simulink model "sampleModel313"  (R2021b)
settings: Solver=VariableStepAuto  StartTime=0.0  StopTime=10.0  RelTol=1e-3
undefined symbols (not defined in the file or in its folder): Newton, Raphson
libraries: simulink x5, slpidlib x1
settings Model: Creator=user  LastModifiedBy=user

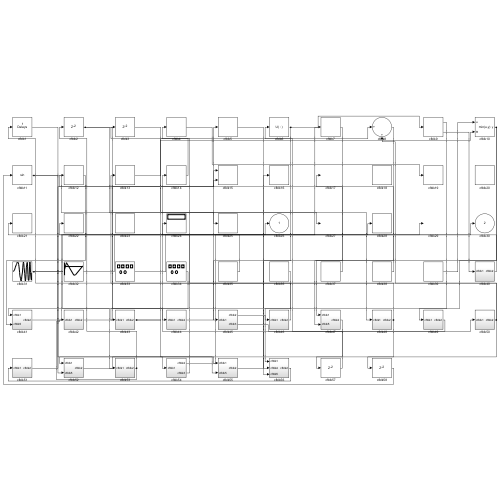
[thumbnail: Simulink's stored preview of the top-level diagram]
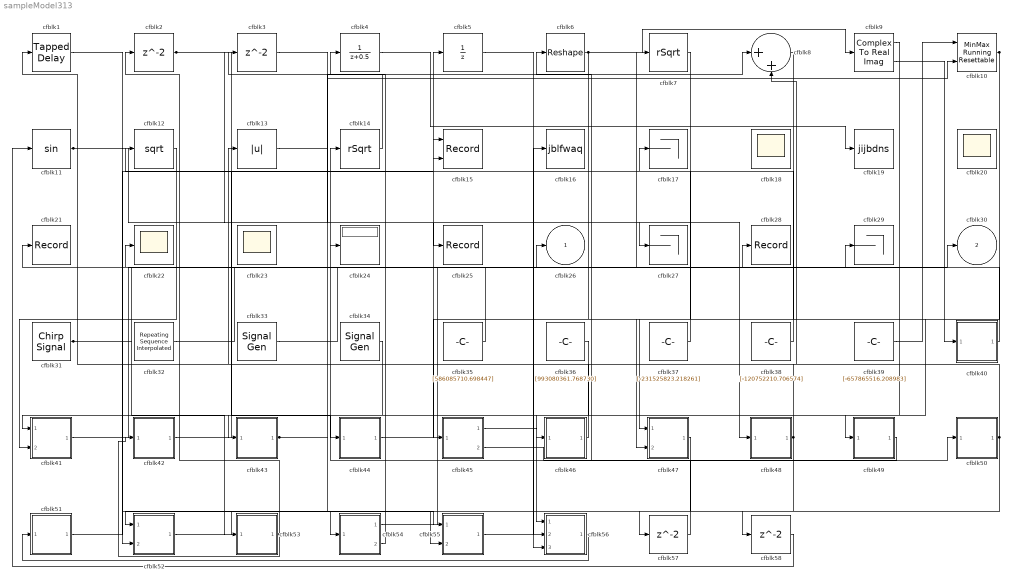
== system sampleModel313 ==
  cfblk1 : simulink/Discrete/Tapped Delay  vinit=0.0  samptime=-1  NumDelays=1  DelayOrder=Oldest  includeCurrent=off
  cfblk10 : simulink/Math Operations/MinMax Running Resettable  Function=min  vinit=0.0
  cfblk11 : Trigonometry
  cfblk12 : Sqrt  SaturateOnIntegerOverflow=on
  cfblk13 : Abs
  cfblk14 : Sqrt  Operator=rSqrt  AlgorithmType=Newton-Raphson  SaturateOnIntegerOverflow=on
  cfblk15 : Record  FileSettingsInternal="{\"entries\":[{\"content\":{\"excelSettings\":{\"content\":{},\"type\":\"Streamout.ExcelSettings\"}},\"type\":\"Streamout.FileSettingStorage\",\"uuid\":\"90899390-830c-4f20-99b3-b71a0b28f61d\"}],\"packageUris\":[\"http://schema.mathworks.com/mf0/streamout_blocks/R2020a\"],\"version\":\"1.0\"}"  Layout=[1 1]  SignalsInternal="{\"entries\":[{\"content\":{\"signals\":[{\"content\":{\"blockPath\":[\"sampleModel313/cfblk15\"],\"channel\":[],\"dimensions\":[1],\"domain\":\"sampleModel313/cfblk15\",\"lineColor\":\"#a2142f\",\"plots\":[1],\"port\":1,\"sid\":[\"\"],\"signalID\":13225,\"signalName\":\"cfblk42\"},\"type\":\"RecordBlkView.Signal\",\"uuid\":\"8692cdac-150e-44d6-933d-60e6954af18a\"},{\"content\":{\"blockPath\":[\"sampleModel313/cfblk15\"],\"channel\":[],\"dimensions\":[1],\"domain\":\"sampleModel313/cfblk15\",\"lineColor\":\"#139fff\",\"plots\":[1],\"port\":2,\"sid\":[\"\"],\"signalID\":13229,\"signalName\":\"cfblk51\"},\"type\":\"RecordBlkView.Signal\",\"uuid\":\"bc72ad84-1dd7-4dd2-a75b-1e74ba305bc3\"}]},\"type\":\"RecordBlkView.InputSignals\",\"uuid\":\"f9261edf-1019-4a70-a12e-24402ee5b183\"}],\"packageUris\":[\"http://schema.mathworks.com/mf0/streamout_blocks/R2020a\"],\"version\":\"1.0\"}"  VisualizationBindings="{\"xyplotplugin\":{\"info\":[{\"series\":[{\"bindingParametersList\":[{\"parameter\":\"X-Axis\",\"signalID\":13225,\"signalName\":\"cfblk42\"},{\"parameter\":\"Y-Axis\",\"signalID\":13229,\"signalName\":\"cfblk51\"}],\"seriesID\":56227}],\"subplotID\":1}]}}"  CompatibilityTag=XY
  cfblk16 : ToWorkspace  VariableName=jblfwaq  SaveFormat=Timeseries  SampleTime=-1
  cfblk17 : Terminator
  cfblk{18,20,22..23} (4 alike) : Scope
      cfblk18 settings: Floating=on
      cfblk20 settings: Floating=on
      cfblk23 settings: Floating=on
  cfblk19 : ToWorkspace  VariableName=jijbdns  SaveFormat=Timeseries  SampleTime=-1
  cfblk{2..3,57..58} (4 alike) : Delay  SampleTime=1
  cfblk21 : Record  FileSettingsInternal="{\"entries\":[{\"content\":{\"excelSettings\":{\"content\":{},\"type\":\"Streamout.ExcelSettings\"}},\"type\":\"Streamout.FileSettingStorage\",\"uuid\":\"64d57652-56fd-4ca2-b7c9-7809ea16690a\"}],\"packageUris\":[\"http://schema.mathworks.com/mf0/streamout_blocks/R2020a\"],\"version\":\"1.0\"}"  SignalsInternal="{\"entries\":[{\"content\":{\"signals\":[{\"content\":{\"blockPath\":[\"sampleModel313/cfblk21\"],\"channel\":[],\"dimensions\":[1],\"domain\":\"sampleModel313/cfblk21\",\"lineColor\":\"#d95319\",\"plots\":[1],\"port\":1,\"sid\":[\"\"],\"signalID\":13233,\"signalName\":\"cfblk54:2\"},\"type\":\"RecordBlkView.Signal\",\"uuid\":\"e54faf43-b919-4a37-b4a8-d819c38ad15e\"}]},\"type\":\"RecordBlkView.InputSignals\",\"uuid\":\"55d9d209-326f-41d9-bd73-887f268fbcdd\"}],\"packageUris\":[\"http://schema.mathworks.com/mf0/streamout_blocks/R2020a\"],\"version\":\"1.0\"}"  VisualizationBindings="{\"sparklinesplugin\":{\"info\":[{\"bindingParametersList\":[],\"subplotID\":1}]}}"
  cfblk24 : Display
  cfblk25 : Record  FileSettingsInternal="{\"entries\":[{\"content\":{\"excelSettings\":{\"content\":{},\"type\":\"Streamout.ExcelSettings\"}},\"type\":\"Streamout.FileSettingStorage\",\"uuid\":\"0e3c709e-7826-4611-a778-3b371a044123\"}],\"packageUris\":[\"http://schema.mathworks.com/mf0/streamout_blocks/R2020a\"],\"version\":\"1.0\"}"  SignalsInternal="{\"entries\":[{\"content\":{\"signals\":[{\"content\":{\"blockPath\":[\"sampleModel313/cfblk25\"],\"channel\":[],\"dimensions\":[1],\"domain\":\"sampleModel313/cfblk25\",\"lineColor\":\"#edb120\",\"plots\":[1],\"port\":1,\"sid\":[\"\"],\"signalID\":13237,\"signalName\":\"cfblk3\"},\"type\":\"RecordBlkView.Signal\",\"uuid\":\"58c6856b-a54d-45f5-97ff-c25ca7fd5d44\"}]},\"type\":\"RecordBlkView.InputSignals\",\"uuid\":\"b6ba7e50-83e3-437d-acd1-c6e268323c3a\"}],\"packageUris\":[\"http://schema.mathworks.com/mf0/streamout_blocks/R2020a\"],\"version\":\"1.0\"}"  VisualizationBindings="{\"sparklinesplugin\":{\"info\":[{\"bindingParametersList\":[],\"subplotID\":1}]}}"
  cfblk27 : Terminator
  cfblk28 : Record  FileSettingsInternal="{\"entries\":[{\"content\":{\"excelSettings\":{\"content\":{},\"type\":\"Streamout.ExcelSettings\"}},\"type\":\"Streamout.FileSettingStorage\",\"uuid\":\"65d362b9-fb87-4f77-ab4e-bc625eaa5118\"}],\"packageUris\":[\"http://schema.mathworks.com/mf0/streamout_blocks/R2020a\"],\"version\":\"1.0\"}"  SignalsInternal="{\"entries\":[{\"content\":{\"signals\":[{\"content\":{\"blockPath\":[\"sampleModel313/cfblk28\"],\"channel\":[],\"dimensions\":[1],\"domain\":\"sampleModel313/cfblk28\",\"lineColor\":\"#7e2f8e\",\"plots\":[1],\"port\":1,\"sid\":[\"\"],\"signalID\":13241,\"signalName\":\"cfblk41\"},\"type\":\"RecordBlkView.Signal\",\"uuid\":\"2a321a31-f066-4655-b88e-f634fd74f6e1\"}]},\"type\":\"RecordBlkView.InputSignals\",\"uuid\":\"8034e422-48cb-4a9f-8c33-6a108b75bc03\"}],\"packageUris\":[\"http://schema.mathworks.com/mf0/streamout_blocks/R2020a\"],\"version\":\"1.0\"}"  VisualizationBindings="{\"sparklinesplugin\":{\"info\":[{\"bindingParametersList\":[],\"subplotID\":1}]}}"
  cfblk29 : Terminator
  cfblk31 : simulink/Sources/Chirp Signal  f1=[-8417458.251595]  T=[-100350191.950646]  f2=[445002722.912709]
  cfblk32 : simulink/Sources/Repeating Sequence Interpolated  OutValues=[-322752428.282228, 451461590.106244, -965527425.871181, -937878614.000823, 66698759.911813]  TimeValues=[0 0.1 0.5 0.6 1].'  LookUpMeth=Interpolation-Use End Values  tsamp=0.01  OutMin=[]  OutMax=[]  OutDataTypeStr=double  OutputDataTypeScalingMode=double  OutDataType=fixdt(0,8)  OutScaling=2^-10
  cfblk33 : SignalGenerator  Amplitude=[-595473010.535318]
  cfblk34 : SignalGenerator  WaveForm=square  Amplitude=[543712172.056688]
  cfblk35 : Constant  Value=[586085710.698447]  SampleTime=1
  cfblk36 : Constant  Value=[993080361.768730]  SampleTime=1
  cfblk37 : Constant  Value=[-231525823.218261]  SampleTime=1
  cfblk38 : Constant  Value=[-120752210.706574]  SampleTime=1
  cfblk39 : Constant  Value=[-657865516.208983]  SampleTime=1
  cfblk4 : DiscreteTransferFcn  SampleTime=1
  cfblk40 : Subsystem
  cfblk41 : Subsystem
  cfblk42 : Subsystem
  cfblk43 : Subsystem
  cfblk44 : Subsystem
  cfblk45 : Subsystem
  cfblk46 : Subsystem
  cfblk47 : Subsystem
  cfblk48 : Subsystem
  cfblk49 : Subsystem
  cfblk5 : UnitDelay  HasFrameUpgradeWarning=on
  cfblk50 : Subsystem
  cfblk51 : Subsystem
  cfblk52 : Subsystem
  cfblk53 : Subsystem
  cfblk54 : Subsystem
  cfblk55 : Subsystem
  cfblk56 : Subsystem
  cfblk6 : Reshape
  cfblk7 : Sqrt  Operator=rSqrt  AlgorithmType=Newton-Raphson  SaturateOnIntegerOverflow=on
  cfblk8 : Sum  Inputs=|++
  cfblk9 : ComplexToRealImag
  cfblk26 : Outport
  cfblk30 : Outport  Port=2
  wires:
  cfblk7/1 -> cfblk47/1(cfblk1)
  cfblk49/1(cfblk2) -> cfblk14/1
  cfblk48/1(cfblk2) -> cfblk1/1, cfblk58/1
  cfblk47/1(cfblk2) -> cfblk52/1(cfblk1)
  cfblk41/1(cfblk2) -> cfblk28/1
  cfblk39/1 -> cfblk10/1
  cfblk37/1 -> cfblk17/1
  cfblk45/1(cfblk2) -> cfblk56/1(cfblk1)
  cfblk10/1 -> cfblk49/1(cfblk1), cfblk47/2(cfblk5)
  cfblk2/1 -> cfblk44/1(cfblk1), cfblk27/1
  cfblk53/1(cfblk2) -> cfblk42/1(cfblk1), cfblk2/1
  cfblk44/1(cfblk2) -> cfblk5/1
  cfblk34/1 -> cfblk41/1(cfblk1)
  cfblk13/1 -> cfblk8/1
  cfblk36/1 -> cfblk46/1(cfblk1)
  cfblk35/1 -> cfblk24/1
  cfblk1/1 -> cfblk52/2(cfblk5)
  cfblk4/1 -> cfblk19/1
  cfblk45/2(cfblk3) -> cfblk50/1(cfblk1)
  cfblk12/1 -> cfblk41/2(cfblk5)
  cfblk40/1(cfblk2) -> cfblk22/1
  cfblk56/1(cfblk2) -> cfblk51/1(cfblk1)
  cfblk5/1 -> cfblk56/2(cfblk4)
  cfblk42/1(cfblk2) -> cfblk15/1
  cfblk6/1 -> cfblk9/1, cfblk45/1(cfblk1)
  cfblk11/1 -> cfblk48/1(cfblk1), cfblk55/1(cfblk1)
  cfblk32/1 -> cfblk26/1
  cfblk50/1(cfblk2) -> cfblk13/1, cfblk8/2, cfblk57/1
  cfblk46/1(cfblk2) -> cfblk4/1
  cfblk51/1(cfblk2) -> cfblk15/2
  cfblk54/1(cfblk2) -> cfblk29/1
  cfblk9/1 -> cfblk43/1(cfblk1)
  cfblk38/1 -> cfblk12/1
  cfblk54/2(cfblk3) -> cfblk21/1
  cfblk8/1 -> cfblk56/3(cfblk5)
  cfblk31/1 -> cfblk16/1, cfblk53/1(cfblk1)
  cfblk55/1(cfblk2) -> cfblk30/1
  cfblk9/2 -> cfblk40/1(cfblk1)
  cfblk3/1 -> cfblk25/1
  cfblk14/1 -> cfblk3/1
  cfblk43/1(cfblk2) -> cfblk10/2, cfblk55/2(cfblk5)
  cfblk52/1(cfblk2) -> cfblk54/1(cfblk1)
  cfblk33/1 -> cfblk7/1
  cfblk57/1 -> cfblk6/1
  cfblk58/1 -> cfblk11/1

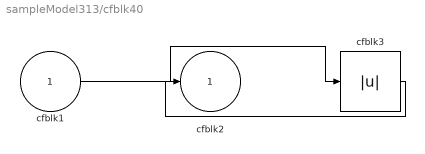
== system sampleModel313/cfblk40 ==
  cfblk1 : Inport
  cfblk3 : Abs
  cfblk2 : Outport
  wires:
  cfblk1/1 -> cfblk3/1
  cfblk3/1 -> cfblk2/1

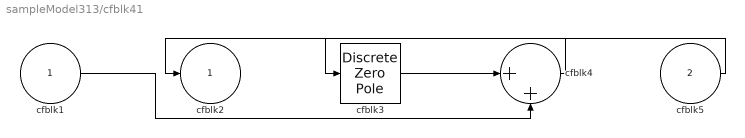
== system sampleModel313/cfblk41 ==
  cfblk1 : Inport
  cfblk5 : Inport  Port=2
  cfblk3 : DiscreteZeroPole  Poles=[0 0.5]  Gain=1
  cfblk4 : Sum  Inputs=|++
  cfblk2 : Outport
  wires:
  cfblk3/1 -> cfblk4/1
  cfblk4/1 -> cfblk2/1
  cfblk1/1 -> cfblk4/2
  cfblk5/1 -> cfblk3/1

== system sampleModel313/cfblk42 ==
  cfblk1 : Inport
  cfblk3 : DiscreteZeroPole  Poles=[0 0.5]  Gain=1
  cfblk2 : Outport
  wires:
  cfblk1/1 -> cfblk3/1
  cfblk3/1 -> cfblk2/1

== system sampleModel313/cfblk43 ==
  cfblk1 : Inport
  cfblk3 : Product  Inputs=**
  cfblk2 : Outport
  wires:
  cfblk3/1 -> cfblk2/1
  cfblk1/1 -> cfblk3/1, cfblk3/2

== system sampleModel313/cfblk44 ==
  cfblk1 : Inport
  cfblk3 : PermuteDimensions
  cfblk2 : Outport
  wires:
  cfblk1/1 -> cfblk3/1
  cfblk3/1 -> cfblk2/1

== system sampleModel313/cfblk45 ==
  cfblk1 : Inport
  cfblk2 : Outport
  cfblk3 : Outport  Port=2
  wires:
  cfblk1/1 -> cfblk2/1, cfblk3/1

== system sampleModel313/cfblk46 ==
  cfblk1 : Inport
  cfblk3 : Sum  Inputs=|++
  cfblk2 : Outport
  wires:
  cfblk1/1 -> cfblk3/1, cfblk3/2
  cfblk3/1 -> cfblk2/1

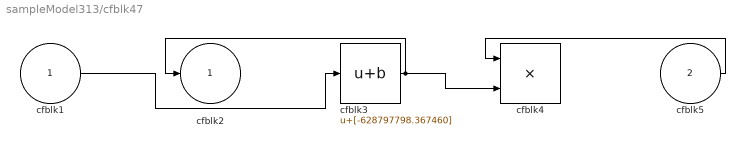
== system sampleModel313/cfblk47 ==
  cfblk1 : Inport
  cfblk5 : Inport  Port=2
  cfblk3 : Bias  Bias=[-628797798.367460]
  cfblk4 : Product  Inputs=**
  cfblk2 : Outport
  wires:
  cfblk3/1 -> cfblk2/1, cfblk4/2
  cfblk1/1 -> cfblk3/1
  cfblk5/1 -> cfblk4/1

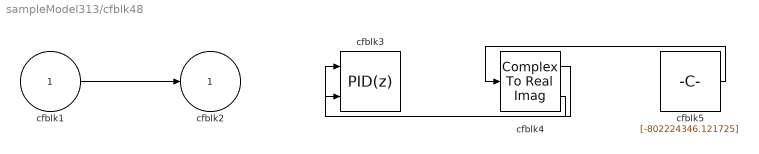
== system sampleModel313/cfblk48 ==
  cfblk1 : Inport
  cfblk3 : slpidlib/PID Controller (2DOF)  Controller=PID  Form=Parallel  TimeDomain=Discrete-time  UseExternalTs=off  SampleTime=1  IntegratorMethod=Forward Euler  FilterMethod=Forward Euler  ControllerParametersSource=internal  P=1  I=1  D=0  UseFilter=on  N=100  b=1  c=1  TunerSelectOption=Transfer Function Based (PID Tuner App)  InitialConditionSource=internal  InitialConditionForIntegrator=0  InitialConditionForFilter=0  DifferentiatorICPrevScaledInput=0  ExternalReset=none  TrackingMode=off  Kt=1  LimitOutput=off  SatLimitsSource=internal  UpperSaturationLimit=inf  LowerSaturationLimit=-inf  LinearizeAsGain=off  AntiWindupMode=none  Kb=1  POutMin=[]  POutMax=[]  IOutMin=[]  IOutMax=[]  DOutMin=[]  DOutMax=[]  NOutMin=[]  NOutMax=[]  bOutMin=[]  bOutMax=[]  cOutMin=[]  cOutMax=[]  SumOutMin=[]  SumOutMax=[]  SaturationOutMin=[]  SaturationOutMax=[]  PParamMin=[]  PParamMax=[]  IParamMin=[]  IParamMax=[]  DParamMin=[]  DParamMax=[]  NParamMin=[]  NParamMax=[]  bParamMin=[]  bParamMax=[]  cParamMin=[]  cParamMax=[]  KbParamMin=[]  KbParamMax=[]  KtParamMin=[]  KtParamMax=[]  KbOutMin=[]  KbOutMax=[]  KtOutMin=[]  KtOutMax=[]  IntegratorOutMin=[]  IntegratorOutMax=[]  FilterOutMin=[]  FilterOutMax=[]  SumI1OutMin=[]  SumI1OutMax=[]  SumI2OutMin=[]  SumI2OutMax=[]  SumI3OutMin=[]  SumI3OutMax=[]  SumI4OutMin=[]  SumI4OutMax=[]  SumDOutMin=[]  SumDOutMax=[]  Sum1OutMin=[]  Sum1OutMax=[]  Sum2OutMin=[]  Sum2OutMax=[]  Sum3OutMin=[]  Sum3OutMax=[]  DifferentiatorOutMin=[]  DifferentiatorOutMax=[]  FilterDiffOutCoefMin=[]  FilterDiffOutCoefMax=[]  ReciprocalOutMin=[]  ReciprocalOutMax=[]  SumDenOutMin=[]  SumDenOutMax=[]  SumNumOutMin=[]  SumNumOutMax=[]  DivideOutMin=[]  DivideOutMax=[]  UdiffTsProdOutMin=[]  UdiffTsProdOutMax=[]  NTsProdOutMin=[]  NTsProdOutMax=[]  UintegralTsProdOutMin=[]  UintegralTsProdOutMax=[]  UngainTsProdOutMin=[]  UngainTsProdOutMax=[]  IntegratorContinuousStateAttributes=''  IntegratorStateMustResolveToSignalObject=off  IntegratorRTWStateStorageClass=Auto  FilterContinuousStateAttributes=''  FilterStateMustResolveToSignalObject=off  FilterRTWStateStorageClass=Auto  ParallelPVariant=InternalParameters  IdealPVariant=Disabled  IVariant=InternalParameters  DVariant=InternalParameters  bVariant=InternalParameters  cVariant=InternalParameters  IntegratorVariant=Discrete  SatVariant=Disabled  AWVariant=Passthrough  PCopyVariant=Disabled  TRVariant=Disabled  FdbkBlocksVariant=Forward  IdealPFdbkVariant=Disabled  SatFdbkVariant=Disabled  DerivativeFilterVariant=ForwardEulerFilter  NVariant=InternalParameters  NCopyVariant=Disabled  FilterICVariant=InternalICsFilter  IntegratorICVariant=InternalICs  ExternalResetVariant=Disabled  TRSumVariant=Passthrough  SumFdbkVariant=Disabled  SumVariant=Sum_PID  TsampFilterVariant=InternalTs  TsampNgainVariant=Passthrough  TsampIntegralVariant=Passthrough  ExternalSaturationOutDataTypeStr=Inherit: Same as second input
      settings: SourceProductBaseCode=SL
  cfblk4 : ComplexToRealImag
  cfblk5 : Constant  Value=[-802224346.121725]  SampleTime=1
  cfblk2 : Outport
  wires:
  cfblk1/1 -> cfblk2/1
  cfblk5/1 -> cfblk4/1
  cfblk4/1 -> cfblk3/1
  cfblk4/2 -> cfblk3/2

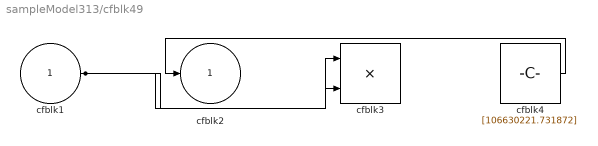
== system sampleModel313/cfblk49 ==
  cfblk1 : Inport
  cfblk3 : Product
  cfblk4 : Constant  Value=[106630221.731872]  SampleTime=1
  cfblk2 : Outport
  wires:
  cfblk4/1 -> cfblk2/1
  cfblk1/1 -> cfblk3/1, cfblk3/2

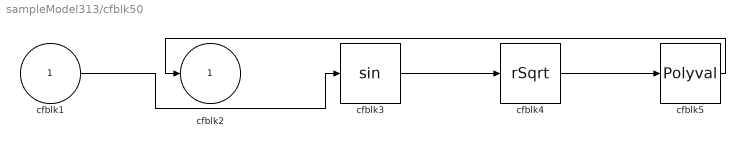
== system sampleModel313/cfblk50 ==
  cfblk1 : Inport
  cfblk3 : Trigonometry
  cfblk4 : Sqrt  Operator=rSqrt  AlgorithmType=Newton-Raphson  SaturateOnIntegerOverflow=on
  cfblk5 : Polyval  Coefs=[ +2.081618890e-019, -1.441693666e-014, +4.719686976e-010, -8.536869453e-006, +1.621573104e-001, -8.087801117e+001 ]
  cfblk2 : Outport
  wires:
  cfblk5/1 -> cfblk2/1
  cfblk3/1 -> cfblk4/1
  cfblk4/1 -> cfblk5/1
  cfblk1/1 -> cfblk3/1

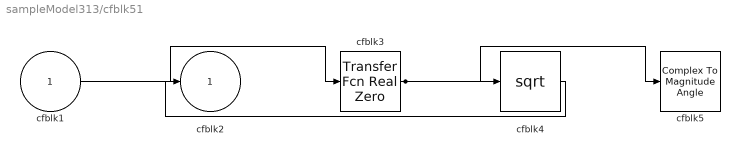
== system sampleModel313/cfblk51 ==
  cfblk1 : Inport
  cfblk3 : simulink/Discrete/Transfer Fcn Real Zero  ZeroZ=0.75  ICPrevInput=0.0  DoSatur=off
      settings: SourceProductBaseCode=SL
  cfblk4 : Sqrt  SaturateOnIntegerOverflow=on
  cfblk5 : ComplexToMagnitudeAngle
  cfblk2 : Outport
  wires:
  cfblk1/1 -> cfblk3/1
  cfblk4/1 -> cfblk2/1
  cfblk3/1 -> cfblk4/1, cfblk5/1

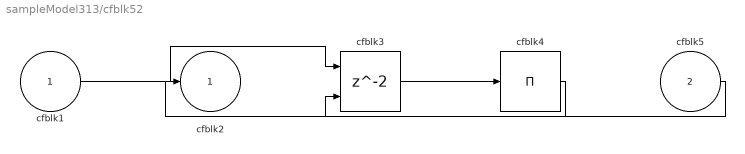
== system sampleModel313/cfblk52 ==
  cfblk1 : Inport
  cfblk5 : Inport  Port=2
  cfblk3 : Delay  ShowEnablePort=on  SampleTime=1
      settings: InputPortMap=u0,e6
  cfblk4 : Product  Inputs=*
  cfblk2 : Outport
  wires:
  cfblk1/1 -> cfblk3/1
  cfblk3/1 -> cfblk4/1
  cfblk4/1 -> cfblk2/1
  cfblk5/1 -> cfblk3/2

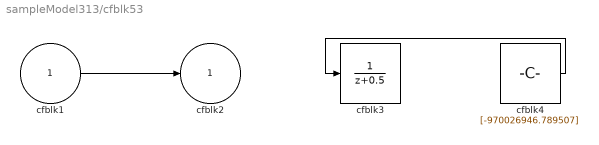
== system sampleModel313/cfblk53 ==
  cfblk1 : Inport
  cfblk3 : DiscreteTransferFcn  SampleTime=1
  cfblk4 : Constant  Value=[-970026946.789507]  SampleTime=1
  cfblk2 : Outport
  wires:
  cfblk4/1 -> cfblk3/1
  cfblk1/1 -> cfblk2/1

== system sampleModel313/cfblk54 ==
  cfblk1 : Inport
  cfblk2 : Outport
  cfblk3 : Outport  Port=2
  wires:
  cfblk1/1 -> cfblk3/1, cfblk2/1

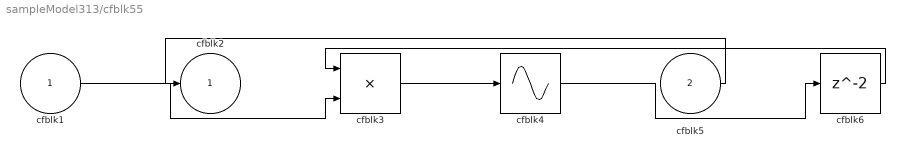
== system sampleModel313/cfblk55 ==
  cfblk1 : Inport
  cfblk5 : Inport  Port=2
  cfblk3 : Product
  cfblk4 : Sin  TimeSource=Use external signal  SampleTime=0
  cfblk6 : Delay  SampleTime=1
  cfblk2 : Outport
  wires:
  cfblk1/1 -> cfblk3/2
  cfblk5/1 -> cfblk2/1
  cfblk3/1 -> cfblk4/1
  cfblk4/1 -> cfblk6/1
  cfblk6/1 -> cfblk3/1

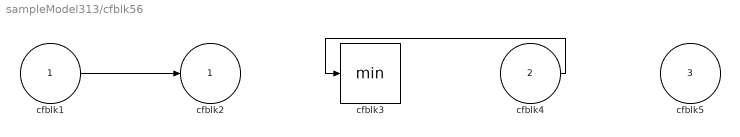
== system sampleModel313/cfblk56 ==
  cfblk1 : Inport
  cfblk4 : Inport  Port=2
  cfblk5 : Inport  Port=3
  cfblk3 : MinMax
  cfblk2 : Outport
  wires:
  cfblk1/1 -> cfblk2/1
  cfblk4/1 -> cfblk3/1
